simulink model "abs_CS9_LDM_w_EBRDBR"  (Simulink 9.2)
settings: Solver=FixedStepAuto  StartTime=0  StopTime=20  FixedStep=0.0005  RelTol=1e-3  AbsTol=1e-6
values from neighbouring files (symbols this model uses):
  K_Cntr_HiSpd_u8 = 10.0    [DBR_V002.sldd]
  K_Cntr_LowSpd_u8 = 10.0    [DBR_V002.sldd]
  K_Cntr_NrmlSpd_u8 = 10.0    [DBR_V002.sldd]
  K_Cntr_Sdstl_u8 = 10.0    [DBR_V002.sldd]
  K_CSTCtol_ramp_lower = -800.0    [DBR_V002.sldd]
  K_CSTCtol_ramp_upper = 800.0    [DBR_V002.sldd]
  K_DBR_aDBRCSTminDecel = 100.0    [DBR_V002.sldd]
  K_DBR_aDBRDecelEmgHigh_CST_u16 = 500.0    [DBR_V002.sldd]
  K_DBR_aDBRDecelSftLow_CST_u16 = 200.0    [DBR_V002.sldd]
  K_DBR_aDBRDecelStdlstlDegdlvl1_u16 = 600.0    [DBR_V002.sldd]
  K_DBR_aDBRDecelStdlstlDegdlvl2_u16 = 1200.0    [DBR_V002.sldd]
  K_DBR_blCSTSwch_bl = 0.0    [DBR_V002.sldd]
  K_DBR_coDBRDecelFactor1 = 5.0    [DBR_V002.sldd]
  K_DBR_coDBRDecelFactor2 = 3.0    [DBR_V002.sldd]
  K_DBR_lenDBRStdlstlDegdlvl_u16 = 1800.0    [DBR_V002.sldd]
  K_DBR_velCSTPdlDistSpdLmt_s16 = 100.0    [DBR_V002.sldd]
  K_DBR_velDBRCSTlowVehSpd_u16 = 8.0    [DBR_V002.sldd]
  K_DBR_velVehSpdLow_CST_s16 = 14.0    [DBR_V002.sldd]
  K_EBR_aACCHold_flat_u16 = 200.0    [DBR_V002.sldd]
  K_EBR_ACC_ramp_lower = -800.0    [DBR_V002.sldd]
  K_EBR_ACC_ramp_upper = 800.0    [DBR_V002.sldd]
  K_EBR_ACCSBDeclEterDecl_u16 = 200.0    [DBR_V002.sldd]
  K_EBR_ACCSBDeclSlope = 1.0    [DBR_V002.sldd]
  K_EBR_ACCSBminDecl = 100.0    [DBR_V002.sldd]
  K_EBR_velACCVehSpdHiLim_u16 = 431.0    [DBR_V002.sldd]
  K_EBR_velACCVehSpdLim_buffer = 1.0    [DBR_V002.sldd]
  K_EBR_velACCVehSpdLoLim_u16 = 14.0    [DBR_V002.sldd]
  W_EBR_velACCSBEntrVehSpd_u16 = 0.0    [DBR_V002.sldd]
undefined symbols (not defined in the file or in its folder): sigbuilder_block
libraries: simulink x8, LDM_Controller x2, Solver_SF x1
(part 2 of 2)

== stateflow chart Get_vehicle_speed_level/Get_vehicle_speed_level ==
  state Over_VehSpd
    en,du:
    V_EBR_stACCVehSpdLvl_en=ACCVehSpdLvl_en_t.over_speed;
  state Normal_VehSpd_To_Over_VehSpd
    en:
    W_Cntr_HiSpd_u8=uint8(0);
    du:
    V_EBR_stACCVehSpdLvl_en=ACCVehSpdLvl_en_t.normal_speed;
    W_Cntr_HiSpd_u8=W_Cntr_HiSpd_u8+1;
  state Over_VehSpd_To_Normal_VehSpd
    en:
    W_Cntr_NrmlSpd_u8=uint8(0);
    du:
    V_EBR_stACCVehSpdLvl_en=ACCVehSpdLvl_en_t.over_speed;
    W_Cntr_NrmlSpd_u8=W_Cntr_NrmlSpd_u8+1;
  state standstill
    en,du:
    V_EBR_stACCVehSpdLvl_en=ACCVehSpdLvl_en_t.standstill;
  state Normal_VehSpd
    en,du:
    V_EBR_stACCVehSpdLvl_en=ACCVehSpdLvl_en_t.normal_speed;
  state standstill_To_Low_VehSpd
    en:
    W_Cntr_LoSpd_u8=uint8(0);
    du:
    V_EBR_stACCVehSpdLvl_en=ACCVehSpdLvl_en_t.standstill;
    W_Cntr_LoSpd_u8=W_Cntr_LoSpd_u8+1;
  state Normal_VehSpd_To_Low_VehSpd
    en:
    W_Cntr_LoSpd_u8=uint8(0);
    du:
    V_EBR_stACCVehSpdLvl_en=ACCVehSpdLvl_en_t.normal_speed;
    W_Cntr_LoSpd_u8=W_Cntr_LoSpd_u8+1;
  state Low_VehSpd_To_Normal_VehSpd
    en:
    W_Cntr_NrmlSpd_u8=uint8(0);
    du:
    V_EBR_stACCVehSpdLvl_en=ACCVehSpdLvl_en_t.low_speed;
    W_Cntr_NrmlSpd_u8=W_Cntr_NrmlSpd_u8+1;
  state Low_VehSpd_To_standstill
    en:
    W_Cntr_StdstlSpd_u8=uint8(0);
    du:
    V_EBR_stACCVehSpdLvl_en=ACCVehSpdLvl_en_t.low_speed;
    W_Cntr_StdstlSpd_u8=W_Cntr_StdstlSpd_u8+1;
  state Low_VehSpd
    en,du:
    V_EBR_stACCVehSpdLvl_en=ACCVehSpdLvl_en_t.low_speed;
  Over_VehSpd -> (junction 119) : [V_DBR_velVehSpd_u16<=K_EBR_velACCVehSpdHiLim_u16-K_EBR_velACCVehSpdLim_buffer]
  (junction 119) -> Over_VehSpd_To_Normal_VehSpd
  (junction 120) -> Over_VehSpd
  Over_VehSpd_To_Normal_VehSpd -> (junction 120) [order 1] : [V_DBR_velVehSpd_u16>K_EBR_velACCVehSpdHiLim_u16+K_EBR_velACCVehSpdLim_buffer]
  (junction 127) -> Over_VehSpd [order 4]
  (junction 121) -> Over_VehSpd
  (junction 122) -> (junction 121) : [W_Cntr_HiSpd_u8>K_Cntr_HiSpd_u8]
  Normal_VehSpd_To_Over_VehSpd -> (junction 122) [order 2]
  (junction 125) -> Normal_VehSpd_To_Over_VehSpd
  Normal_VehSpd_To_Over_VehSpd -> (junction 123) [order 1] : [V_DBR_velVehSpd_u16<=K_EBR_velACCVehSpdHiLim_u16-K_EBR_velACCVehSpdLim_buffer]
  Over_VehSpd_To_Normal_VehSpd -> Normal_VehSpd [order 2] : [W_Cntr_NrmlSpd_u8>K_Cntr_NrmlSpd_u8]
  (junction 123) -> (junction 124)
  (junction 124) -> Normal_VehSpd
  (junction 126) -> (junction 125)
  Normal_VehSpd -> (junction 126) [order 1] : [V_DBR_velVehSpd_u16>K_EBR_velACCVehSpdHiLim_u16+K_EBR_velACCVehSpdLim_buffer]
  (default) -> (junction 127)
  (junction 127) -> standstill [order 3] : [V_DBR_velVehSpd_u16==uint16(0)]
  (junction 127) -> Normal_VehSpd [order 1] : [V_DBR_velVehSpd_u16<=K_EBR_velACCVehSpdHiLim_u16&&V_DBR_velVehSpd_u16>K_EBR_velACCVehSpdLoLim_u16]
  (junction 127) -> Low_VehSpd [order 2] : [V_DBR_velVehSpd_u16<=K_EBR_velACCVehSpdLoLim_u16]
  standstill -> (junction 128) : [V_DBR_velVehSpd_u16>K_EBR_velACCVehSpdLim_buffer]
  (junction 128) -> standstill_To_Low_VehSpd
  (junction 129) -> Normal_VehSpd
  Low_VehSpd_To_Normal_VehSpd -> (junction 129) [order 1] : [W_Cntr_NrmlSpd_u8>K_Cntr_NrmlSpd_u8]
  Normal_VehSpd -> Normal_VehSpd_To_Low_VehSpd [order 2] : [V_DBR_velVehSpd_u16<=K_EBR_velACCVehSpdLoLim_u16-K_EBR_velACCVehSpdLim_buffer]
  Normal_VehSpd_To_Low_VehSpd -> Normal_VehSpd [order 1] : [V_DBR_velVehSpd_u16>K_EBR_velACCVehSpdLoLim_u16+K_EBR_velACCVehSpdLim_buffer]
  (junction 130) -> standstill : [V_DBR_velVehSpd_u16==uint16(0)]
  standstill_To_Low_VehSpd -> (junction 130) [order 1]
  Low_VehSpd_To_standstill -> standstill [order 2] : [W_Cntr_StdstlSpd_u8>K_Cntr_Sdstl_u8]
  standstill_To_Low_VehSpd -> (junction 131) [order 2] : [W_Cntr_LoSpd_u8>K_Cntr_LowSpd_u8]
  (junction 131) -> Low_VehSpd
  Normal_VehSpd_To_Low_VehSpd -> (junction 136) [order 2] : [W_Cntr_LoSpd_u8>K_Cntr_LowSpd_u8]
  Low_VehSpd_To_Normal_VehSpd -> (junction 133) [order 2] : [V_DBR_velVehSpd_u16<=K_EBR_velACCVehSpdLoLim_u16-K_EBR_velACCVehSpdLim_buffer]
  (junction 135) -> Low_VehSpd_To_Normal_VehSpd
  (junction 133) -> (junction 132)
  (junction 132) -> Low_VehSpd
  Low_VehSpd_To_standstill -> (junction 137) [order 1]
  (junction 134) -> Low_VehSpd_To_standstill
  Low_VehSpd -> (junction 134) [order 2] : [V_DBR_velVehSpd_u16==uint16(0)]
  Low_VehSpd -> (junction 135) [order 1] : [V_DBR_velVehSpd_u16>K_EBR_velACCVehSpdLoLim_u16+K_EBR_velACCVehSpdLim_buffer]
  (junction 136) -> Low_VehSpd
  (junction 137) -> Low_VehSpd : [V_DBR_velVehSpd_u16<K_EBR_velACCVehSpdLim_buffer&&...
      | V_DBR_velVehSpd_u16>0]
  data: V_DBR_velVehSpd_u16 input uint16; V_EBR_stACCVehSpdLvl_en output Enum: ACCVehSpdLvl_en_t; K_EBR_velACCVehSpdHiLim_u16 parameter uint16; K_EBR_velACCVehSpdLoLim_u16 parameter uint16; K_Cntr_HiSpd_u8 parameter uint8; K_Cntr_LowSpd_u8 parameter uint8; K_Cntr_Sdstl_u8 parameter uint8; K_EBR_velACCVehSpdLim_buffer parameter uint16; K_Cntr_NrmlSpd_u8 parameter uint8; W_Cntr_HiSpd_u8 local uint8; W_Cntr_NrmlSpd_u8 local uint8; W_Cntr_LoSpd_u8 local uint8; W_Cntr_StdstlSpd_u8 local uint8

== stateflow chart ACC/ACC ==
  state ACC_off
    en,du:
    V_EBR_aCHACCDecelReq_u16=uint16(0);
    V_EBR_stCHACCRunbleSts_en=CHACCRunbleSts_en_t.ACC_off;
    V_EBR_stCHACCEPBReq_en=CHACCEPBReq_en_t.no_request;
    ACC_off -> (junction 191) [order 1]
    (junction 191) -> (junction 190) [order 1] : [V_EBR_stACCFalCseSts_en==ACCFalCseSts_en_t.fail_cause1]
    (junction 191) -> (junction 192) [order 2] : [V_EBR_stACCFalCseSts_en==ACCFalCseSts_en_t.fail_cause2||...
        | V_EBR_stACCFalCseSts_en==ACCFalCseSts_en_t.fail_cause3||...
        | V_EBR_stACCFalCseSts_en==ACCFalCseSts_en_t.fail_cause4]
    (junction 190) -> (junction 194) : {V_EBR_stACCResp_en=ACCResp_en_t.precondition_not_satisfied;}
    (junction 191) -> (junction 193) [order 3]
    (junction 192) -> (junction 196) : {V_EBR_stACCResp_en=ACCResp_en_t.control_not_allowed;}
    (junction 193) -> (junction 195) : {V_EBR_stACCResp_en=ACCResp_en_t.no_request;}
    (junction 194) -> (junction 195)
    (junction 196) -> (junction 195)
  state ACC_standby
    en,du:
    V_EBR_aCHACCDecelReq_u16=uint16(0);
    V_EBR_stCHACCRunbleSts_en=CHACCRunbleSts_en_t.ACC_standby;
    (junction 207) -> (junction 206) [order 1] : [V_DBR_EBR_stBrkArbMode_en~=BrkArbMode_en_t.ACC_arbitration]
    ACC_standby -> (junction 207) [order 1]
    (junction 206) -> (junction 211) : {V_EBR_stACCResp_en=ACCResp_en_t.lost_arbitration;...
        | V_EBR_stCHACCEPBReq_en=CHACCEPBReq_en_t.no_request;}
    (junction 207) -> (junction 209) [order 2]
    (junction 209) -> (junction 208) [order 3]
    (junction 209) -> (junction 210) [order 1] : [V_EBR_stACCFalCseSts_en==ACCFalCseSts_en_t.fail_cause1]
    (junction 210) -> (junction 213) : {V_EBR_stACCResp_en=ACCResp_en_t.precondition_not_satisfied;...
        | V_EBR_stCHACCEPBReq_en=CHACCEPBReq_en_t.no_request;}
    (junction 208) -> (junction 213) : {V_EBR_stACCResp_en=ACCResp_en_t.request_honoured;...
        | V_EBR_stCHACCEPBReq_en=CHACCEPBReq_en_t.no_request;}
    (junction 209) -> (junction 212) [order 2] : [V_EBR_stACCFalCseSts_en==ACCFalCseSts_en_t.fail_cause2||...
        | V_EBR_stACCFalCseSts_en==ACCFalCseSts_en_t.fail_cause3||...
        | V_EBR_stACCFalCseSts_en==ACCFalCseSts_en_t.fail_cause4]
    (junction 211) -> (junction 214)
    (junction 212) -> (junction 213) : {V_EBR_stACCResp_en=ACCResp_en_t.control_not_allowed;...
        | V_EBR_stCHACCEPBReq_en=CHACCEPBReq_en_t.no_request;}
    (junction 214) -> (junction 213)
  state ACC_control_brake
    en,du:
    V_EBR_aCHACCDecelReq_u16=V_EBR_aACCReqValue_u16;
    V_EBR_stCHACCRunbleSts_en=CHACCRunbleSts_en_t.ACC_CB;
    V_EBR_stACCResp_en=ACCResp_en_t.request_honoured;
    V_EBR_stCHACCEPBReq_en=CHACCEPBReq_en_t.no_request;
  state ACC_self_brake
    en,du:
    V_EBR_stCHACCRunbleSts_en=CHACCRunbleSts_en_t.ACC_CB;
    V_EBR_stACCResp_en=ACCResp_en_t.request_honoured;
    V_EBR_stCHACCEPBReq_en=CHACCEPBReq_en_t.no_request;
    ACC_self_brake -> (junction 227) [order 1]
    (junction 227) -> (junction 228) [order 1] : [W_EBR_ACC_SB_flag_bl==false]
    (junction 228) -> (junction 229) : {W_EBR_ACC_SB_decel_s16=V_VDS_aACCLong_s16;...
        | W_EBR_velACCSBEntrVehSpd_u16=V_DBR_velVehSpd_s16;}
    (junction 227) -> (junction 230) [order 2]
    (junction 229) -> (junction 232) : {V_EBR_aCHACCDecelReq_u16=ACC_SB_curve1(V_DBR_velVehSpd_s16,W_EBR_ACC_SB_decel_s16);}
    (junction 230) -> (junction 231) : {W_EBR_velACCSBEntrVehSpd_u16=V_DBR_velVehSpd_s16;}
    (junction 231) -> (junction 232) : {V_EBR_aCHACCDecelReq_u16=ACC_SB_curve2(V_DBR_velVehSpd_s16);}
  state ACC_EPB
    en:
    V_EBR_stCHACCEPBReq_en=CHACCEPBReq_en_t.apply_request;
    du:
    V_EBR_stCHACCRunbleSts_en=CHACCRunbleSts_en_t.ACC_EPB;
    V_EBR_stACCResp_en=ACCResp_en_t.request_honoured;
    ex:
    V_EBR_aCHACCDecelReq_u16=uint16(0);
  state ACC_hold
    en,du:
    V_EBR_aCHACCDecelReq_u16=ACC_hold_curve(V_VDS_degRdSlopeLong_s16);
    V_EBR_stCHACCRunbleSts_en=CHACCRunbleSts_en_t.ACC_HOLD;
    V_EBR_stACCResp_en=ACCResp_en_t.request_honoured;
    V_EBR_stCHACCEPBReq_en=CHACCEPBReq_en_t.no_request;
  state V_EBR_aCHACCDecelReq_u16=ACC_SB_curve1(V_DBR_velVehSpd_s16,W_EBR_ACC_SB_decel_s16) [function]
  state V_EBR_aCHACCDecelReq_u16=ACC_SB_curve2(V_DBR_velVehSpd_s16) [function]
  state V_EBR_aCHACCDecelReq_u16=ACC_hold_curve(V_VDS_degRdSlopeLong_s16) [function]
  (default) -> ACC_off
  ACC_off -> ACC_standby [order 1] : [V_EBR_stACCFalCseSts_en==ACCFalCseSts_en_t.no_error&&...
      | (V_EBR_stACCSysSts_en==ACCSysSts_en_t.active||...
      | V_EBR_stACCSysSts_en==ACCSysSts_en_t.brake_only)]
  ACC_standby -> ACC_off [order 1] : [V_EBR_stACCEPBSts_en==ACCEPBSts_en_t.apply || V_EBR_stACCStdbySkpSts_en==ACCStdbySkpSts_en_t.off]
  ACC_hold -> ACC_standby [order 2] : [V_EBR_stACCHldSkpSts_en==ACCHldSkpSts_en_t.standby...
      | ||V_DBR_EBR_stBrkArbMode_en~=BrkArbMode_en_t.ACC_arbitration]
  ACC_standby -> ACC_self_brake [order 3] : [V_EBR_stACCStdbySkpSts_en==ACCStdbySkpSts_en_t.self_brake...
      | &&V_DBR_EBR_stBrkArbMode_en==BrkArbMode_en_t.ACC_arbitration]...
      | {W_EBR_ACC_SB_flag_bl=true;}
  ACC_EPB -> ACC_standby : [V_EBR_stACCEPBSts_en==ACCEPBSts_en_t.apply]
  ACC_self_brake -> ACC_standby [order 3] : [V_EBR_stACCBrkSkpSts_en==ACCBrkSkpSts_en_t.standby...
      | || V_DBR_EBR_stBrkArbMode_en~=BrkArbMode_en_t.ACC_arbitration]
  ACC_standby -> ACC_control_brake [order 2] : [V_EBR_stACCStdbySkpSts_en==ACCStdbySkpSts_en_t.control_brake...
      | &&V_DBR_EBR_stBrkArbMode_en==BrkArbMode_en_t.ACC_arbitration]
  ACC_control_brake -> ACC_standby [order 1] : [V_EBR_stACCBrkSkpSts_en==ACCBrkSkpSts_en_t.standby...
      | ||V_DBR_EBR_stBrkArbMode_en~=BrkArbMode_en_t.ACC_arbitration]
  ACC_control_brake -> ACC_self_brake [order 2] : [V_EBR_stACCBrkSkpSts_en==ACCBrkSkpSts_en_t.self_brake...
      | &&V_DBR_EBR_stBrkArbMode_en==BrkArbMode_en_t.ACC_arbitration]...
      | {W_EBR_ACC_SB_flag_bl=false;}
  ACC_self_brake -> ACC_control_brake [order 1] : [V_EBR_stACCBrkSkpSts_en==ACCBrkSkpSts_en_t.control_brake...
      | &&V_DBR_EBR_stBrkArbMode_en==BrkArbMode_en_t.ACC_arbitration]
  ACC_hold -> ACC_EPB [order 1] : [(V_EBR_stACCSebltSts_en~=ACCSebltSts_en_t.wear_seat_belt ||...
      | V_EBR_stACCDrvrDorOpnSts_en ~= ACCDrvrDorOpnSts_en_t.closed||...
      | V_EBR_stACCHldSkpSts_en==ACCHldSkpSts_en_t.EPB)...
      | &&K_EBR_blACCEPBSwch_bl==true]
  ACC_control_brake -> ACC_hold [order 3] : [V_EBR_stACCBrkSkpSts_en==ACCBrkSkpSts_en_t.hold...
      | &&V_DBR_EBR_stBrkArbMode_en==BrkArbMode_en_t.ACC_arbitration]
  ACC_self_brake -> ACC_hold [order 2] : [V_EBR_stACCBrkSkpSts_en==ACCBrkSkpSts_en_t.hold...
      | &&V_DBR_EBR_stBrkArbMode_en==BrkArbMode_en_t.ACC_arbitration]
  data: V_DBR_velVehSpd_s16 function_input int16 size=1; W_EBR_ACC_SB_decel_s16 function_input int16 size=1; V_EBR_aCHACCDecelReq_u16 function_output double; V_DBR_velVehSpd_s16 function_input int16 size=1; V_EBR_aCHACCDecelReq_u16 function_output double; V_VDS_degRdSlopeLong_s16 function_input int16 size=1; V_EBR_aCHACCDecelReq_u16 function_output double; V_DBR_EBR_stBrkArbMode_en input Enum: BrkArbMode_en_t; V_EBR_stACCStdbySkpSts_en input Enum: ACCStdbySkpSts_en_t; V_EBR_stACCBrkSkpSts_en input Enum: ACCBrkSkpSts_en_t; V_EBR_stACCHldSkpSts_en input Enum: ACCHldSkpSts_en_t; V_EBR_stACCFalCseSts_en input Enum: ACCFalCseSts_en_t; V_EBR_stACCSysSts_en input Enum: ACCSysSts_en_t; V_EBR_stACCEPBSts_en input Enum: ACCEPBSts_en_t; V_EBR_aACCReqValue_u16 input uint16; V_EBR_stACCSebltSts_en input Enum: ACCSebltSts_en_t; V_EBR_stACCDrvrDorOpnSts_en input Enum: ACCDrvrDorOpnSts_en_t; V_VDS_degRdSlopeLong_s16 input int16; V_VDS_aACCLong_s16 input int16; V_DBR_velVehSpd_s16 input int16; V_EBR_aCHACCDecelReq_u16 output uint16; V_EBR_stCHACCRunbleSts_en output Enum: CHACCRunbleSts_en_t; V_EBR_stACCResp_en output Enum: ACCResp_en_t; V_EBR_stCHACCEPBReq_en output Enum: CHACCEPBReq_en_t; W_EBR_ACC_SB_flag_bl local boolean; W_EBR_ACC_SB_decel_s16 local int16; K_EBR_blACCEPBSwch_bl parameter boolean; W_EBR_velACCSBEntrVehSpd_u16 local int16
